simulink model "rlc_notch_electrical"  (R2020a)
settings: Solver=FixedStepAuto  StartTime=0.0  StopTime=duration  FixedStep=deltaT  RelTol=1e-3
values from neighbouring files (symbols this model uses):
  A = 1    [dataAnalisys.m]
  C = 1000*1e-6    (= 0.001)    [dataAnalisys.m]
  deltaT = 2*pi/(w*m)    [dataAnalisys.m]
  L = 1000*1e-3    (= 1)    [dataAnalisys.m]
  R = 1    [dataAnalisys.m]
  w = omega(i)    [dataAnalisys.m]
libraries: powerlib x7
settings Model: Creator=acer  LastModifiedBy=acer

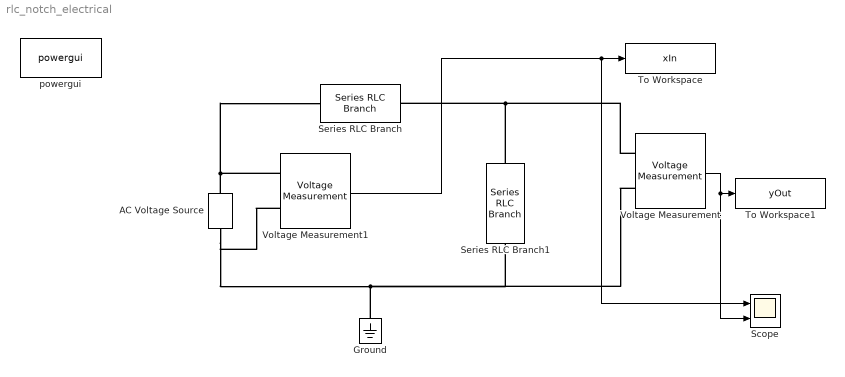
== system rlc_notch_electrical ==
  AC Voltage Source : powerlib/Electrical Sources/AC Voltage Source  Amplitude=A  Phase=0  Frequency=w/(2*pi)  SampleTime=-1  Measurements=None  BusType=swing  Pref=10e3  Qref=0  Qmin=-inf  Qmax=+inf
  Ground : powerlib/Elements/Ground  LConnTagsString=a
  Scope : Scope  NumInputPorts=2
  Series RLC Branch : powerlib/Elements/Series RLC Branch  LConnTagsString=__new0  RConnTagsString=__new0  BranchType=R  Resistance=R  Inductance=1e-3  SetiL0=off  InitialCurrent=0  Capacitance=1e-6  Setx0=off  InitialVoltage=0  Measurements=None
  Series RLC Branch1 : powerlib/Elements/Series RLC Branch  LConnTagsString=__new0  RConnTagsString=__new0  BranchType=LC  Resistance=1  Inductance=L  SetiL0=off  InitialCurrent=0  Capacitance=C  Setx0=off  InitialVoltage=0  Measurements=None
  To Workspace : ToWorkspace  VariableName=xIn  SampleTime=-1
      settings: Save2DSignal=2-D array (concatenate along first dimension)
  To Workspace1 : ToWorkspace  VariableName=yOut  SampleTime=-1
      settings: Save2DSignal=2-D array (concatenate along first dimension)
  Voltage Measurement : powerlib/Measurements/Voltage Measurement  PhasorSimulation=off  OutputType=Complex  PSBequivalent=0
  Voltage Measurement1 : powerlib/Measurements/Voltage Measurement  PhasorSimulation=off  OutputType=Complex  PSBequivalent=0
  powergui : powerlib/powergui  Priority=1  SimulationMode=Discrete  SampleTime=deltaT  frequency=60  Iterations=50  frequencyindice=5.02929620170389  Pbase=100e6  ErrMax=1e-4  UnitsV=kV  UnitsW=MW  buscounter=0  FunctionMessages=off  echomessages=off  EnableUseOfTLC=off  CurrentSourceSwitches=off  DisableSnubberDevices=off  DisableRonSwitches=off  DisableVfSwitches=off  DisplayEquations=off  AutomaticDiscreteSolvers=off  SolverType=Tustin/Backward Euler (TBE)  Interpol=off  ExternalGateDelay=off  methode=off  Ts=100  x0status=blocks  SPID=on  SwTol=0  HookPort=off  NonlinearTolerance=1e-4  nMaxIteration=100  ContinueOnMaxIteration=off  RestoreLinks=warning  ResistiveCurrentMeasurement=off  Frange=[0:2:500]  Ylog=off  Xlog=on  ShowGrid=off  save=off  variable=ZData  structure=0  ZoomFFT=off  StartTime=0.0  cycles=1  DisplayStyle=1  fundamental=60  FreqAxis=off  MaxFrequency=1000  frequencyindicesteady=1  RmsSteady=1  display=off
  wires:
  Voltage Measurement1/1 -> Scope/1, To Workspace/1
  Voltage Measurement/1 -> Scope/2, To Workspace1/1
  connections:
  Series RLC Branch1/LConn1 -- Series RLC Branch/RConn1 -- Voltage Measurement/LConn1
  AC Voltage Source/RConn1 -- Series RLC Branch/LConn1 -- Voltage Measurement1/LConn1
  Ground/LConn1 -- Series RLC Branch1/RConn1 -- Voltage Measurement/LConn2 -- Voltage Measurement1/LConn2 -- AC Voltage Source/LConn1
